simulink model "Regler_Kaskadierung_2_PID"  (R2017b)
settings: Solver=FixedStepAuto  StartTime=0.0  StopTime=20000  FixedStep=0.5  RelTol=1e-3
undefined symbols (not defined in the file or in its folder): K_M, Kd_S, Ki_S, Kp_S, Tt_S
libraries: cstblocks x2, simulink x1
settings Model: Creator=arbno  LastModifiedBy=arbno

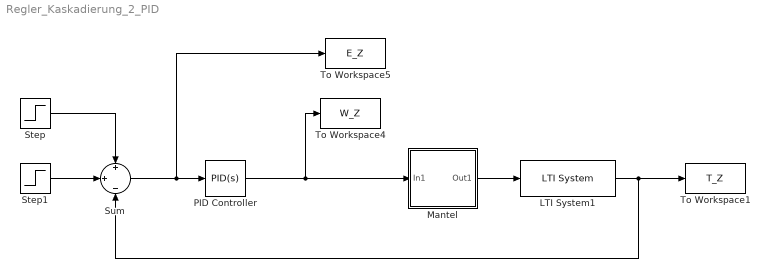
== system Regler_Kaskadierung_2_PID ==
  LTI System1 : cstblocks/LTI System  sys=G_Zelle  IC=[]
  Mantel : Subsystem
  PID Controller : simulink/Continuous/PID Controller  Controller=PID  TimeDomain=Continuous-time  SampleTime=-1  IntegratorMethod=Forward Euler  FilterMethod=Forward Euler  Form=Parallel  UseFilter=on  ControllerParametersSource=internal  P=Kp_S  I=Ki_S  D=Kd_S  N=0.3  InitialConditionSource=internal  InitialConditionForIntegrator=0  InitialConditionForFilter=0  ExternalReset=none  LimitOutput=on  UpperSaturationLimit=141  LowerSaturationLimit=0  LinearizeAsGain=on  AntiWindupMode=back-calculation  Kb=1/Tt_S  TrackingMode=off  Kt=1  PParamMin=[]  PParamMax=[]  IParamMin=[]  IParamMax=[]  DParamMin=[]  DParamMax=[]  NParamMin=[]  NParamMax=[]  KbParamMin=[]  KbParamMax=[]  KtParamMin=[]  KtParamMax=[]  POutMin=[]  POutMax=[]  IOutMin=[]  IOutMax=[]  DOutMin=[]  DOutMax=[]  NOutMin=[]  NOutMax=[]  KbOutMin=[]  KbOutMax=[]  KtOutMin=[]  KtOutMax=[]  IntegratorOutMin=[]  IntegratorOutMax=[]  FilterOutMin=[]  FilterOutMax=[]  SumOutMin=[]  SumOutMax=[]  SumI1OutMin=[]  SumI1OutMax=[]  SumI2OutMin=[]  SumI2OutMax=[]  SumI3OutMin=[]  SumI3OutMax=[]  SumDOutMin=[]  SumDOutMax=[]  SaturationOutMin=[]  SaturationOutMax=[]  IntegratorContinuousStateAttributes=''  IntegratorStateMustResolveToSignalObject=off  IntegratorRTWStateStorageClass=Auto  FilterContinuousStateAttributes=''  FilterStateMustResolveToSignalObject=off  FilterRTWStateStorageClass=Auto  DifferentiatorICPrevScaledInput=0  DifferentiatorOutMin=[]  DifferentiatorOutMax=[]  InitialConditionSetting=State (most efficient)  FilterDiffOutCoefMin=[]  FilterDiffOutCoefMax=[]  SumDenOutMin=[]  SumDenOutMax=[]  SumNumOutMin=[]  SumNumOutMax=[]  ReciprocalOutMin=[]  ReciprocalOutMax=[]  DivideOutMin=[]  DivideOutMax=[]  TunerSelectOption=Transfer Function Based (PID Tuner App)
  Step : Step  Time=0  After=80  SampleTime=0
  Step1 : Step  Time=0  After=0  SampleTime=0
  Sum : Sum  Inputs=+|+|-
  To Workspace1 : ToWorkspace  VariableName=T_Z  SaveFormat=Structure With Time  SampleTime=-1
  To Workspace4 : ToWorkspace  VariableName=W_Z  SaveFormat=Structure With Time  SampleTime=-1
  To Workspace5 : ToWorkspace  VariableName=E_Z  SaveFormat=Structure With Time  SampleTime=-1
  wires:
  Mantel/1(Out1) -> LTI System1/1
  LTI System1/1 -> To Workspace1/1, Sum/3
  Step/1 -> Sum/1
  Sum/1 -> To Workspace5/1, PID Controller/1
  Step1/1 -> Sum/2
  PID Controller/1 -> Mantel/1(In1), To Workspace4/1

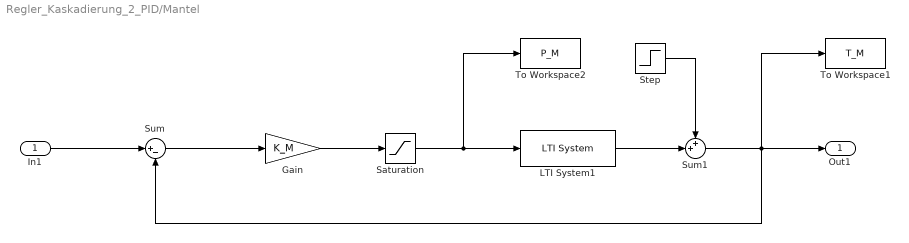
== system Regler_Kaskadierung_2_PID/Mantel ==
  In1 : Inport
  Gain : Gain  Gain=K_M
  LTI System1 : cstblocks/LTI System  sys=G_Mantel  IC=[]
  Saturation : Saturate  UpperLimit=1  LowerLimit=0
  Step : Step  Time=12000  After=10  SampleTime=0
  Sum : Sum  Inputs=|+-
  Sum1 : Sum  Inputs=++|
  To Workspace1 : ToWorkspace  VariableName=T_M  SaveFormat=Structure With Time  SampleTime=-1
  To Workspace2 : ToWorkspace  VariableName=P_M  SaveFormat=Structure With Time  SampleTime=-1
  Out1 : Outport
  wires:
  LTI System1/1 -> Sum1/2
  Sum/1 -> Gain/1
  In1/1 -> Sum/1
  Gain/1 -> Saturation/1
  Saturation/1 -> LTI System1/1, To Workspace2/1
  Sum1/1 -> Sum/2, To Workspace1/1, Out1/1
  Step/1 -> Sum1/1
